simulink model "ISC_V1"  (R2017b)
settings: Solver=VariableStepAuto  StartTime=0.0  StopTime=10.0  RelTol=1e-3
undefined symbols (not defined in the file or in its folder): par
settings Model: Creator=gdgra  LastModifiedBy=gdgra

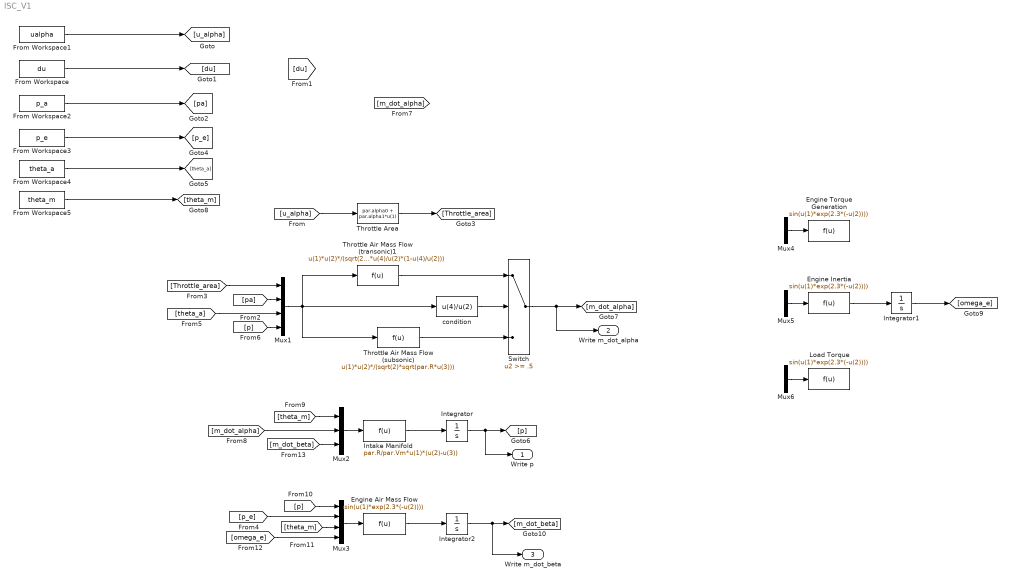
== system ISC_V1 ==
  Engine Air Mass Flow : Fcn  Expr=sin(u(1)*exp(2.3*(-u(2))))
  Engine Inertia : Fcn  Expr=sin(u(1)*exp(2.3*(-u(2))))
  Engine Torque Generation : Fcn  Expr=sin(u(1)*exp(2.3*(-u(2))))
  From Workspace : FromWorkspace  VariableName=du  SampleTime=0
  From Workspace1 : FromWorkspace  VariableName=ualpha  SampleTime=0
  From Workspace2 : FromWorkspace  VariableName=p_a  SampleTime=0
  From Workspace3 : FromWorkspace  VariableName=p_e  SampleTime=0
  From Workspace4 : FromWorkspace  VariableName=theta_a  SampleTime=0
  From Workspace5 : FromWorkspace  VariableName=theta_m  SampleTime=0
  Intake Manifold : Fcn  Expr=par.R/par.Vm*u(1)*(u(2)-u(3))
  Integrator : Integrator
  Integrator1 : Integrator
  Integrator2 : Integrator
  Load Torque : Fcn  Expr=sin(u(1)*exp(2.3*(-u(2))))
  Mux1 : Mux
  Mux2 : Mux  Inputs=3
  Mux3 : Mux
  Mux4 : Mux  Inputs=2
  Mux5 : Mux  Inputs=2
  Mux6 : Mux  Inputs=2
  Switch : Switch  Threshold=.5
  Throttle Air Mass Flow (subsonic) : Fcn  Expr=u(1)*u(2)*/(sqrt(2)*sqrt(par.R*u(3)))
  Throttle Air Mass Flow (transonic)1 : Fcn  Expr=u(1)*u(2)*/(sqrt(2)*sqrt(par.R*u(3)))*sqrt(2*u(4)/u(2)*(1-u(4)/u(2)))
  Throttle Area : Fcn  Expr=par.alpha0 + par.alpha1*u(1)
  "condition " : Fcn  Expr=u(4)/u(2)
  Write p : Outport
  Write m_dot_alpha : Outport  Port=2
  Write m_dot_beta : Outport  Port=3
  wires:
  From Workspace1/1 -> [u_alpha]
  From Workspace/1 -> [du]
  From Workspace2/1 -> [pa]
  [u_alpha] -> Throttle Area/1
  Mux2/1 -> Intake Manifold/1
  Mux3/1 -> Engine Air Mass Flow/1
  Mux4/1 -> Engine Torque Generation/1
  Mux5/1 -> Engine Inertia/1
  Mux6/1 -> Load Torque/1
  Throttle Area/1 -> [Throttle_area]
  [Throttle_area] -> Mux1/1
  From Workspace3/1 -> [p_e]
  From Workspace4/1 -> [theta_a]
  [pa] -> Mux1/2
  [theta_a] -> Mux1/3
  Intake Manifold/1 -> Integrator/1
  Integrator/1 -> Write p/1, [p]
  [p] -> Mux1/4
  Throttle Air Mass Flow (subsonic)/1 -> Switch/3
  Mux1/1 -> Throttle Air Mass Flow (transonic)1/1, Throttle Air Mass Flow (subsonic)/1, "condition "/1
  "condition "/1 -> Switch/2
  Throttle Air Mass Flow (transonic)1/1 -> Switch/1
  Switch/1 -> Write m_dot_alpha/1, [m_dot_alpha]
  [m_dot_alpha] -> Mux2/2
  From Workspace5/1 -> [theta_m]
  [theta_m] -> Mux2/1
  [p] -> Mux3/1
  [p_e] -> Mux3/2
  [theta_m] -> Mux3/3
  Engine Inertia/1 -> Integrator1/1
  Integrator1/1 -> [omega_e]
  [omega_e] -> Mux3/4
  Engine Air Mass Flow/1 -> Integrator2/1
  Integrator2/1 -> Write m_dot_beta/1, [m_dot_beta]
  [m_dot_beta] -> Mux2/3
